simulink model "Blank_SS_only_ABC"  (R2018b)
settings: Solver=VariableStepAuto  StartTime=0.0  StopTime=10  RelTol=1e-3
undefined symbols (not defined in the file): A, B, C, D
settings Model: Creator=Johan PC  LastModifiedBy=Johan PC

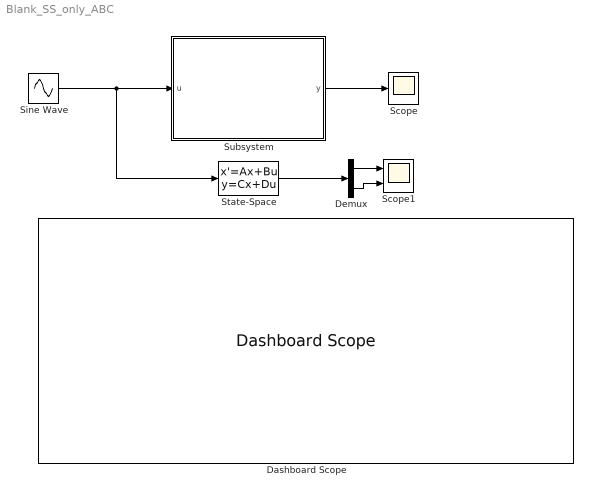
== system Blank_SS_only_ABC ==
  Dashboard Scope : DashboardScope  WebBlockId=19
  Demux : Demux  Outputs=2
  Scope : Scope
  Scope1 : Scope  NumInputPorts=2
  Sine Wave : Sin  Amplitude=0.30  Frequency=0.5  SampleTime=0
  State-Space : StateSpace  A=A  B=B  C=C  D=D  InitialCondition=0
  Subsystem : Subsystem
  wires:
  Sine Wave/1 -> State-Space/1, Subsystem/1(u)
  Subsystem/1(y) -> Scope/1
  State-Space/1 -> Demux/1
  Demux/1 -> Scope1/1
  Demux/2 -> Scope1/2

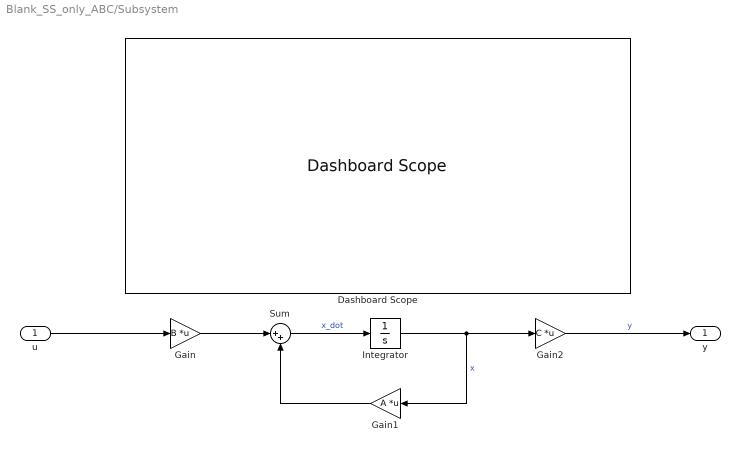
== system Blank_SS_only_ABC/Subsystem ==
  u : Inport
  Dashboard Scope : DashboardScope  WebBlockId=20
  Gain : Gain  Gain=B  Multiplication=Matrix(K*u)
  Gain1 : Gain  Gain=A  Multiplication=Matrix(K*u)
  Gain2 : Gain  Gain=C  Multiplication=Matrix(K*u)
  Integrator : Integrator
  Sum : Sum  Inputs=|++
  y : Outport
  wires:
  u/1 -> Gain/1
  Gain2/1 -> y/1  "y"
  Integrator/1 -> Gain1/1, Gain2/1  "x"
  Gain/1 -> Sum/1
  Sum/1 -> Integrator/1  "x_dot"
  Gain1/1 -> Sum/2
